simulink model "Xe_Model_Redo_June_26"  (R2018a)
settings: Solver=VariableStepAuto  StartTime=0.0  StopTime=5E5+96*60*60  RelTol=1e-3
values from neighbouring files (symbols this model uses):
  A_pipe = pi*r_pipe^2    (= 0.0126676869774)    [Startup_Script.m]
  alpha_FS = 0.517E-16    (= 5.17e-17)    [Startup_Script.m]
  alpha_G_R1 = 0.334E-17    (= 3.34e-18)    [Startup_Script.m]
  alpha_G_R2 = 0.699E-17    (= 6.99e-18)    [Startup_Script.m]
  alpha_G_R3 = 0.669E-17    (= 6.69e-18)    [Startup_Script.m]
  alpha_G_R4 = 0.791E-18    (= 7.91e-19)    [Startup_Script.m]
  D_g = 2.37E-9    (= 2.37e-09)    [Startup_Script.m]
  epsilon = 0.1    [Startup_Script.m]
  eta_b = 1E-4    (= 0.0001)    [Startup_Script.m]
  eta_fs = 1.2E-4    (= 0.00012)    [Startup_Script.m]
  f_cv = 0.004    [Startup_Script.m]
  FS_Mu_A = 4340    [Startup_Script.m]
  FS_Mu_K = 0.084    [Startup_Script.m]
  FS_Mu_MSRE = 0.007027    [Startup_Script.m]
  FS_rho_A = 3.628    [Startup_Script.m]
  FS_rho_B = 0.00066    [Startup_Script.m]
  FS_rho_MSRE = 2082    [Startup_Script.m]
  gamma_i = 0.0293524    [Startup_Script.m]
  gamma_te = 0.0322482    [Startup_Script.m]
  gamma_xe = 0.00257324    [Startup_Script.m]
  h_fc = 1.6    [Startup_Script.m]
  H_Xe_a = 5.713e-13    [Startup_Script.m]
  H_Xe_b = -7.937e-10    [Startup_Script.m]
  H_Xe_c = 2.809e-07    [Startup_Script.m]
  HX_r_Tube = ((0.5-0.042)/2)*2.54E-2    (= 0.0058166)    [Startup_Script.m]
  HX_XS = HX_N_Tubes*(pi*HX_r_Tube^2)    (= 0.0168999490356)    [Startup_Script.m]
  k_b = 1.3806E-23    (= 1.3806e-23)    [Startup_Script.m]
  lambda_i = 2.9306070546251702E-5    (= 2.93060705463e-05)    [Startup_Script.m]
  lambda_te = 0.036481430555786593    (= 0.0364814305558)    [Startup_Script.m]
  lambda_xe = 2.0924e-05    [Startup_Script.m]
  N_FC_R1 = 12    [Startup_Script.m]
  N_FC_R2 = 940    [Startup_Script.m]
  N_FC_R3 = 108    [Startup_Script.m]
  N_FC_R4 = 78    [Startup_Script.m]
  P_pump = 35420    [Startup_Script.m]
  phi0 = 3.98E+17    (= 3.98e+17)    [Startup_Script.m]
  phi_G_R_1 = mean(interp1(phi_G_R,phi_G_phi, linspace(0,r_g_r1)))    [Startup_Script.m]
  phi_G_R_2 = mean(interp1(phi_G_R,phi_G_phi, linspace(r_g_r1,r_g_r2)))    [Startup_Script.m]
  phi_G_R_3 = mean(interp1(phi_G_R,phi_G_phi, linspace(r_g_r2,r_g_r3)))    [Startup_Script.m]
  phi_G_R_4 = mean(interp1(phi_G_R,phi_G_phi, linspace(r_g_r3,r_g_r4)))    [Startup_Script.m]
  Q_strpr = 0.003155    [Startup_Script.m]
  Q_tot = 0.07571    [Startup_Script.m]
  r_b = 0.000254    [Startup_Script.m]
  r_fc = 0.79e-2    (= 0.0079)    [Startup_Script.m]
  r_pipe = (5E-2*2.54)/2    (= 0.0635)    [Startup_Script.m]
  r_xe = 2.16E-10    (= 2.16e-10)    [Startup_Script.m]
  Re_CA = 25800    [Startup_Script.m]
  Re_LH = 1E4    (= 10000)    [Startup_Script.m]
  Re_UH = 1E4    (= 10000)    [Startup_Script.m]
  sig_a_xe = 1.18E-22    (= 1.18e-22)    [Startup_Script.m]
  Sig_f = 0.15    [Startup_Script.m]
  T_CA_0 = T_INLET    (= 907.594444444)    [Startup_Script.m]
  T_FP_0 = T_OUTLET    (= 935.372222222)    [Startup_Script.m]
  T_FS_R_1_0 = mean(interp1(R_fs_m,T_fs_K, linspace(0,r_g_r1)))    [Startup_Script.m]
  T_FS_R_2_0 = mean(interp1(R_fs_m,T_fs_K, linspace(r_g_r1,r_g_r2)))    [Startup_Script.m]
  T_FS_R_3_0 = mean(interp1(R_fs_m,T_fs_K, linspace(r_g_r2,r_g_r3)))    [Startup_Script.m]
  T_FS_R_4_0 = mean(interp1(R_fs_m,T_fs_K, linspace(r_g_r3,r_g_r4)))    [Startup_Script.m]
  T_G_R_1_0 = mean(interp1(R_gr_m,T_gr_K, linspace(0,r_g_r1)))    [Startup_Script.m]
  T_HX_0 = 0.5*(T_OUTLET + T_INLET)    (= 921.483333333)    [Startup_Script.m]
  T_LH_0 = T_INLET    (= 907.594444444)    [Startup_Script.m]
  T_Mes = 928.15    [Startup_Script.m]
  T_P100_0 = T_OUTLET    (= 935.372222222)    [Startup_Script.m]
  T_P101_0 = T_OUTLET    (= 935.372222222)    [Startup_Script.m]
  T_P102_0 = T_INLET    (= 907.594444444)    [Startup_Script.m]
  T_Salt_0 = 900    [Startup_Script.m]
  T_UH_0 = T_OUTLET    (= 935.372222222)    [Startup_Script.m]
  U_FC_R1 = 0.607    [Startup_Script.m]
  U_FC_R2 = 0.183    [Startup_Script.m]
  U_FC_R3 = 0.454    [Startup_Script.m]
  U_FC_R4 = 0.250    (= 0.25)    [Startup_Script.m]
  V_CA_0 = 9.7*cubed_foot_to_cubed_meter    (= 0.274673445)    [Startup_Script.m]
  V_FP_0 = (0.9+3.2)*cubed_foot_to_cubed_meter    (= 0.116099085)    [Startup_Script.m]
  V_HX_0 = 6.1*cubed_foot_to_cubed_meter    (= 0.172732785)    [Startup_Script.m]
  V_LH_0 = 10.0*cubed_foot_to_cubed_meter    (= 0.2831685)    [Startup_Script.m]
  V_P100_0 = 2.1*cubed_foot_to_cubed_meter    (= 0.059465385)    [Startup_Script.m]
  V_P101_0 = 0.8*cubed_foot_to_cubed_meter    (= 0.02265348)    [Startup_Script.m]
  V_P102_0 = 2.2*cubed_foot_to_cubed_meter    (= 0.06229707)    [Startup_Script.m]
  V_R1_0 = V_Core_FS_0 *N_FC_R1/N_FC_tot    (= 0.00753107712766)    [Startup_Script.m]
  V_R2_0 = V_Core_FS_0 *N_FC_R2/N_FC_tot    (= 0.589934375)    [Startup_Script.m]
  V_R3_0 = V_Core_FS_0 *N_FC_R3/N_FC_tot    (= 0.0677796941489)    [Startup_Script.m]
  V_R4_0 = V_Core_FS_0 *N_FC_R4/N_FC_tot    (= 0.0489520013298)    [Startup_Script.m]
  V_UH_0 = 10.5*cubed_foot_to_cubed_meter    (= 0.297326925)    [Startup_Script.m]
undefined symbols (not defined in the file or in its folder): magnitude, V_CA, V_HX, V_P2, V_P3, V_R1, V_R2, V_R3, V_R4, V_UH
libraries: simulink x4, dspindex x4, dspstat3 x4, SignalEditorBlockLib x2
(part 11 of 11)

== system Xe_Model_Redo_June_26/Bubbles/Bubble Mass Transfer/Bubble Total KMA/KMA_LH/MTC LH/Re_Num  Scaled/Density W Scaling1/Cantor F1 Density1 ==
  note: K -> deg. C
  T_Salt [k] : Inport
  Constant : Constant  Value=FS_rho_A
  Constant1 : Constant  Value=FS_rho_B
  Constant2 : Constant  Value=273.15
  Display : Display
      settings: Format=short_e
  Display1 : Display
  Product : Product
  Sum : Sum  Inputs=|+-
  Sum1 : Sum  Inputs=+-
  "g/cm^3 -> kg/m^3" : Gain  Gain=1000
  rho [kg/m^3] : Outport
  wires:
  Sum/1 -> "g/cm^3 -> kg/m^3"/1
  Product/1 -> Sum/2
  Constant1/1 -> Display/1, Product/1
  "g/cm^3 -> kg/m^3"/1 -> rho [kg/m^3]/1
  Constant/1 -> Display1/1, Sum/1
  T_Salt [k]/1 -> Sum1/1
  Constant2/1 -> Sum1/2
  Sum1/1 -> Product/2

== system Xe_Model_Redo_June_26/Bubbles/Bubble Mass Transfer/Bubble Total KMA/KMA_LH/MTC LH/Re_Num  Scaled/Density W Scaling3/Cantor F1 Density ==
  note: K -> deg. C
  T_Salt [k] : Inport
  Constant : Constant  Value=FS_rho_A
  Constant1 : Constant  Value=FS_rho_B
  Constant2 : Constant  Value=273.15
  Display : Display
      settings: Format=short_e
  Display1 : Display
  Product : Product
  Sum : Sum  Inputs=|+-
  Sum1 : Sum  Inputs=+-
  "g/cm^3 -> kg/m^3" : Gain  Gain=1000
  rho [kg/m^3] : Outport
  wires:
  Sum/1 -> "g/cm^3 -> kg/m^3"/1
  Product/1 -> Sum/2
  Constant1/1 -> Display/1, Product/1
  "g/cm^3 -> kg/m^3"/1 -> rho [kg/m^3]/1
  Constant/1 -> Display1/1, Sum/1
  T_Salt [k]/1 -> Sum1/1
  Constant2/1 -> Sum1/2
  Sum1/1 -> Product/2

== system Xe_Model_Redo_June_26/Bubbles/Bubble Mass Transfer/Bubble Total KMA/KMA_LH/MTC LH/Re_Num  Scaled/Density W Scaling3/Cantor F1 Density1 ==
  note: K -> deg. C
  T_Salt [k] : Inport
  Constant : Constant  Value=FS_rho_A
  Constant1 : Constant  Value=FS_rho_B
  Constant2 : Constant  Value=273.15
  Display : Display
      settings: Format=short_e
  Display1 : Display
  Product : Product
  Sum : Sum  Inputs=|+-
  Sum1 : Sum  Inputs=+-
  "g/cm^3 -> kg/m^3" : Gain  Gain=1000
  rho [kg/m^3] : Outport
  wires:
  Sum/1 -> "g/cm^3 -> kg/m^3"/1
  Product/1 -> Sum/2
  Constant1/1 -> Display/1, Product/1
  "g/cm^3 -> kg/m^3"/1 -> rho [kg/m^3]/1
  Constant/1 -> Display1/1, Sum/1
  T_Salt [k]/1 -> Sum1/1
  Constant2/1 -> Sum1/2
  Sum1/1 -> Product/2

== system Xe_Model_Redo_June_26/Bubbles/Bubble Mass Transfer/Bubble Total KMA/KMA_LH/MTC LH/Re_Num  Scaled/Viscosity W Scaling1/Cantor Viscosity F1 ==
  T_Salt [k] : Inport
  Constant : Constant  Value=FS_Mu_A
  Constant1 : Constant  Value=FS_Mu_K
  Display1 : Display
  Divide : Product  Inputs=*/
  Math Function : Math  SaturateOnIntegerOverflow=on
  Product : Product
  "centipoise -> Pa S" : Gain  Gain=0.001
  Mu [Pa S] : Outport
  wires:
  Constant1/1 -> Product/2
  T_Salt [k]/1 -> Divide/2
  "centipoise -> Pa S"/1 -> Display1/1, Mu [Pa S]/1
  Product/1 -> "centipoise -> Pa S"/1
  Constant/1 -> Divide/1
  Math Function/1 -> Product/1
  Divide/1 -> Math Function/1

== system Xe_Model_Redo_June_26/Bubbles/Bubble Mass Transfer/Bubble Total KMA/KMA_LH/MTC LH/Re_Num  Scaled/Viscosity W Scaling1/Nominal Value for Cantor Viscosity F1 ==
  T_Salt [k] : Inport
  Constant : Constant  Value=FS_Mu_A
  Constant1 : Constant  Value=FS_Mu_K
  Display1 : Display
  Divide : Product  Inputs=*/
  Math Function : Math  SaturateOnIntegerOverflow=on
  Product : Product
  "centipoise -> Pa S" : Gain  Gain=0.001
  Mu [Pa S] : Outport
  wires:
  Constant1/1 -> Product/2
  T_Salt [k]/1 -> Divide/2
  "centipoise -> Pa S"/1 -> Display1/1, Mu [Pa S]/1
  Product/1 -> "centipoise -> Pa S"/1
  Constant/1 -> Divide/1
  Math Function/1 -> Product/1
  Divide/1 -> Math Function/1

== system Xe_Model_Redo_June_26/Bubbles/Bubble Mass Transfer/Bubble Total KMA/KMA_LH/MTC LH/Re_Num  Scaled/Viscosity W Scaling3/Cantor Viscosity F1 ==
  T_Salt [k] : Inport
  Constant : Constant  Value=FS_Mu_A
  Constant1 : Constant  Value=FS_Mu_K
  Display1 : Display
  Divide : Product  Inputs=*/
  Math Function : Math  SaturateOnIntegerOverflow=on
  Product : Product
  "centipoise -> Pa S" : Gain  Gain=0.001
  Mu [Pa S] : Outport
  wires:
  Constant1/1 -> Product/2
  T_Salt [k]/1 -> Divide/2
  "centipoise -> Pa S"/1 -> Display1/1, Mu [Pa S]/1
  Product/1 -> "centipoise -> Pa S"/1
  Constant/1 -> Divide/1
  Math Function/1 -> Product/1
  Divide/1 -> Math Function/1

== system Xe_Model_Redo_June_26/Bubbles/Bubble Mass Transfer/Bubble Total KMA/KMA_LH/MTC LH/Re_Num  Scaled/Viscosity W Scaling3/Nominal Value for Cantor Viscosity F1 ==
  T_Salt [k] : Inport
  Constant : Constant  Value=FS_Mu_A
  Constant1 : Constant  Value=FS_Mu_K
  Display1 : Display
  Divide : Product  Inputs=*/
  Math Function : Math  SaturateOnIntegerOverflow=on
  Product : Product
  "centipoise -> Pa S" : Gain  Gain=0.001
  Mu [Pa S] : Outport
  wires:
  Constant1/1 -> Product/2
  T_Salt [k]/1 -> Divide/2
  "centipoise -> Pa S"/1 -> Display1/1, Mu [Pa S]/1
  Product/1 -> "centipoise -> Pa S"/1
  Constant/1 -> Divide/1
  Math Function/1 -> Product/1
  Divide/1 -> Math Function/1

== system Xe_Model_Redo_June_26/Bubbles/Bubble Mass Transfer/Bubble Total KMA/KMA_UH/MTC UH/Re_Num  Scaled/Density W Scaling1/Cantor F1 Density ==
  note: K -> deg. C
  T_Salt [k] : Inport
  Constant : Constant  Value=FS_rho_A
  Constant1 : Constant  Value=FS_rho_B
  Constant2 : Constant  Value=273.15
  Display : Display
      settings: Format=short_e
  Display1 : Display
  Product : Product
  Sum : Sum  Inputs=|+-
  Sum1 : Sum  Inputs=+-
  "g/cm^3 -> kg/m^3" : Gain  Gain=1000
  rho [kg/m^3] : Outport
  wires:
  Sum/1 -> "g/cm^3 -> kg/m^3"/1
  Product/1 -> Sum/2
  Constant1/1 -> Display/1, Product/1
  "g/cm^3 -> kg/m^3"/1 -> rho [kg/m^3]/1
  Constant/1 -> Display1/1, Sum/1
  T_Salt [k]/1 -> Sum1/1
  Constant2/1 -> Sum1/2
  Sum1/1 -> Product/2

== system Xe_Model_Redo_June_26/Bubbles/Bubble Mass Transfer/Bubble Total KMA/KMA_UH/MTC UH/Re_Num  Scaled/Density W Scaling1/Cantor F1 Density1 ==
  note: K -> deg. C
  T_Salt [k] : Inport
  Constant : Constant  Value=FS_rho_A
  Constant1 : Constant  Value=FS_rho_B
  Constant2 : Constant  Value=273.15
  Display : Display
      settings: Format=short_e
  Display1 : Display
  Product : Product
  Sum : Sum  Inputs=|+-
  Sum1 : Sum  Inputs=+-
  "g/cm^3 -> kg/m^3" : Gain  Gain=1000
  rho [kg/m^3] : Outport
  wires:
  Sum/1 -> "g/cm^3 -> kg/m^3"/1
  Product/1 -> Sum/2
  Constant1/1 -> Display/1, Product/1
  "g/cm^3 -> kg/m^3"/1 -> rho [kg/m^3]/1
  Constant/1 -> Display1/1, Sum/1
  T_Salt [k]/1 -> Sum1/1
  Constant2/1 -> Sum1/2
  Sum1/1 -> Product/2

== system Xe_Model_Redo_June_26/Bubbles/Bubble Mass Transfer/Bubble Total KMA/KMA_UH/MTC UH/Re_Num  Scaled/Density W Scaling3/Cantor F1 Density ==
  note: K -> deg. C
  T_Salt [k] : Inport
  Constant : Constant  Value=FS_rho_A
  Constant1 : Constant  Value=FS_rho_B
  Constant2 : Constant  Value=273.15
  Display : Display
      settings: Format=short_e
  Display1 : Display
  Product : Product
  Sum : Sum  Inputs=|+-
  Sum1 : Sum  Inputs=+-
  "g/cm^3 -> kg/m^3" : Gain  Gain=1000
  rho [kg/m^3] : Outport
  wires:
  Sum/1 -> "g/cm^3 -> kg/m^3"/1
  Product/1 -> Sum/2
  Constant1/1 -> Display/1, Product/1
  "g/cm^3 -> kg/m^3"/1 -> rho [kg/m^3]/1
  Constant/1 -> Display1/1, Sum/1
  T_Salt [k]/1 -> Sum1/1
  Constant2/1 -> Sum1/2
  Sum1/1 -> Product/2

== system Xe_Model_Redo_June_26/Bubbles/Bubble Mass Transfer/Bubble Total KMA/KMA_UH/MTC UH/Re_Num  Scaled/Density W Scaling3/Cantor F1 Density1 ==
  note: K -> deg. C
  T_Salt [k] : Inport
  Constant : Constant  Value=FS_rho_A
  Constant1 : Constant  Value=FS_rho_B
  Constant2 : Constant  Value=273.15
  Display : Display
      settings: Format=short_e
  Display1 : Display
  Product : Product
  Sum : Sum  Inputs=|+-
  Sum1 : Sum  Inputs=+-
  "g/cm^3 -> kg/m^3" : Gain  Gain=1000
  rho [kg/m^3] : Outport
  wires:
  Sum/1 -> "g/cm^3 -> kg/m^3"/1
  Product/1 -> Sum/2
  Constant1/1 -> Display/1, Product/1
  "g/cm^3 -> kg/m^3"/1 -> rho [kg/m^3]/1
  Constant/1 -> Display1/1, Sum/1
  T_Salt [k]/1 -> Sum1/1
  Constant2/1 -> Sum1/2
  Sum1/1 -> Product/2

== system Xe_Model_Redo_June_26/Bubbles/Bubble Mass Transfer/Bubble Total KMA/KMA_UH/MTC UH/Re_Num  Scaled/Viscosity W Scaling1/Cantor Viscosity F1 ==
  T_Salt [k] : Inport
  Constant : Constant  Value=FS_Mu_A
  Constant1 : Constant  Value=FS_Mu_K
  Display1 : Display
  Divide : Product  Inputs=*/
  Math Function : Math  SaturateOnIntegerOverflow=on
  Product : Product
  "centipoise -> Pa S" : Gain  Gain=0.001
  Mu [Pa S] : Outport
  wires:
  Constant1/1 -> Product/2
  T_Salt [k]/1 -> Divide/2
  "centipoise -> Pa S"/1 -> Display1/1, Mu [Pa S]/1
  Product/1 -> "centipoise -> Pa S"/1
  Constant/1 -> Divide/1
  Math Function/1 -> Product/1
  Divide/1 -> Math Function/1

== system Xe_Model_Redo_June_26/Bubbles/Bubble Mass Transfer/Bubble Total KMA/KMA_UH/MTC UH/Re_Num  Scaled/Viscosity W Scaling1/Nominal Value for Cantor Viscosity F1 ==
  T_Salt [k] : Inport
  Constant : Constant  Value=FS_Mu_A
  Constant1 : Constant  Value=FS_Mu_K
  Display1 : Display
  Divide : Product  Inputs=*/
  Math Function : Math  SaturateOnIntegerOverflow=on
  Product : Product
  "centipoise -> Pa S" : Gain  Gain=0.001
  Mu [Pa S] : Outport
  wires:
  Constant1/1 -> Product/2
  T_Salt [k]/1 -> Divide/2
  "centipoise -> Pa S"/1 -> Display1/1, Mu [Pa S]/1
  Product/1 -> "centipoise -> Pa S"/1
  Constant/1 -> Divide/1
  Math Function/1 -> Product/1
  Divide/1 -> Math Function/1

== system Xe_Model_Redo_June_26/Bubbles/Bubble Mass Transfer/Bubble Total KMA/KMA_UH/MTC UH/Re_Num  Scaled/Viscosity W Scaling3/Cantor Viscosity F1 ==
  T_Salt [k] : Inport
  Constant : Constant  Value=FS_Mu_A
  Constant1 : Constant  Value=FS_Mu_K
  Display1 : Display
  Divide : Product  Inputs=*/
  Math Function : Math  SaturateOnIntegerOverflow=on
  Product : Product
  "centipoise -> Pa S" : Gain  Gain=0.001
  Mu [Pa S] : Outport
  wires:
  Constant1/1 -> Product/2
  T_Salt [k]/1 -> Divide/2
  "centipoise -> Pa S"/1 -> Display1/1, Mu [Pa S]/1
  Product/1 -> "centipoise -> Pa S"/1
  Constant/1 -> Divide/1
  Math Function/1 -> Product/1
  Divide/1 -> Math Function/1

== system Xe_Model_Redo_June_26/Bubbles/Bubble Mass Transfer/Bubble Total KMA/KMA_UH/MTC UH/Re_Num  Scaled/Viscosity W Scaling3/Nominal Value for Cantor Viscosity F1 ==
  T_Salt [k] : Inport
  Constant : Constant  Value=FS_Mu_A
  Constant1 : Constant  Value=FS_Mu_K
  Display1 : Display
  Divide : Product  Inputs=*/
  Math Function : Math  SaturateOnIntegerOverflow=on
  Product : Product
  "centipoise -> Pa S" : Gain  Gain=0.001
  Mu [Pa S] : Outport
  wires:
  Constant1/1 -> Product/2
  T_Salt [k]/1 -> Divide/2
  "centipoise -> Pa S"/1 -> Display1/1, Mu [Pa S]/1
  Product/1 -> "centipoise -> Pa S"/1
  Constant/1 -> Divide/1
  Math Function/1 -> Product/1
  Divide/1 -> Math Function/1

== system Xe_Model_Redo_June_26/Bubbles/Bubble Mass Transfer/CA/KMA_CA/CA  MTC/Re_Num  Scaled/Density W Scaling1/Cantor F1 Density ==
  note: K -> deg. C
  T_Salt [k] : Inport
  Constant : Constant  Value=FS_rho_A
  Constant1 : Constant  Value=FS_rho_B
  Constant2 : Constant  Value=273.15
  Display : Display
      settings: Format=short_e
  Display1 : Display
  Product : Product
  Sum : Sum  Inputs=|+-
  Sum1 : Sum  Inputs=+-
  "g/cm^3 -> kg/m^3" : Gain  Gain=1000
  rho [kg/m^3] : Outport
  wires:
  Sum/1 -> "g/cm^3 -> kg/m^3"/1
  Product/1 -> Sum/2
  Constant1/1 -> Display/1, Product/1
  "g/cm^3 -> kg/m^3"/1 -> rho [kg/m^3]/1
  Constant/1 -> Display1/1, Sum/1
  T_Salt [k]/1 -> Sum1/1
  Constant2/1 -> Sum1/2
  Sum1/1 -> Product/2

== system Xe_Model_Redo_June_26/Bubbles/Bubble Mass Transfer/CA/KMA_CA/CA  MTC/Re_Num  Scaled/Density W Scaling1/Cantor F1 Density1 ==
  note: K -> deg. C
  T_Salt [k] : Inport
  Constant : Constant  Value=FS_rho_A
  Constant1 : Constant  Value=FS_rho_B
  Constant2 : Constant  Value=273.15
  Display : Display
      settings: Format=short_e
  Display1 : Display
  Product : Product
  Sum : Sum  Inputs=|+-
  Sum1 : Sum  Inputs=+-
  "g/cm^3 -> kg/m^3" : Gain  Gain=1000
  rho [kg/m^3] : Outport
  wires:
  Sum/1 -> "g/cm^3 -> kg/m^3"/1
  Product/1 -> Sum/2
  Constant1/1 -> Display/1, Product/1
  "g/cm^3 -> kg/m^3"/1 -> rho [kg/m^3]/1
  Constant/1 -> Display1/1, Sum/1
  T_Salt [k]/1 -> Sum1/1
  Constant2/1 -> Sum1/2
  Sum1/1 -> Product/2

== system Xe_Model_Redo_June_26/Bubbles/Bubble Mass Transfer/CA/KMA_CA/CA  MTC/Re_Num  Scaled/Density W Scaling3/Cantor F1 Density ==
  note: K -> deg. C
  T_Salt [k] : Inport
  Constant : Constant  Value=FS_rho_A
  Constant1 : Constant  Value=FS_rho_B
  Constant2 : Constant  Value=273.15
  Display : Display
      settings: Format=short_e
  Display1 : Display
  Product : Product
  Sum : Sum  Inputs=|+-
  Sum1 : Sum  Inputs=+-
  "g/cm^3 -> kg/m^3" : Gain  Gain=1000
  rho [kg/m^3] : Outport
  wires:
  Sum/1 -> "g/cm^3 -> kg/m^3"/1
  Product/1 -> Sum/2
  Constant1/1 -> Display/1, Product/1
  "g/cm^3 -> kg/m^3"/1 -> rho [kg/m^3]/1
  Constant/1 -> Display1/1, Sum/1
  T_Salt [k]/1 -> Sum1/1
  Constant2/1 -> Sum1/2
  Sum1/1 -> Product/2

== system Xe_Model_Redo_June_26/Bubbles/Bubble Mass Transfer/CA/KMA_CA/CA  MTC/Re_Num  Scaled/Density W Scaling3/Cantor F1 Density1 ==
  note: K -> deg. C
  T_Salt [k] : Inport
  Constant : Constant  Value=FS_rho_A
  Constant1 : Constant  Value=FS_rho_B
  Constant2 : Constant  Value=273.15
  Display : Display
      settings: Format=short_e
  Display1 : Display
  Product : Product
  Sum : Sum  Inputs=|+-
  Sum1 : Sum  Inputs=+-
  "g/cm^3 -> kg/m^3" : Gain  Gain=1000
  rho [kg/m^3] : Outport
  wires:
  Sum/1 -> "g/cm^3 -> kg/m^3"/1
  Product/1 -> Sum/2
  Constant1/1 -> Display/1, Product/1
  "g/cm^3 -> kg/m^3"/1 -> rho [kg/m^3]/1
  Constant/1 -> Display1/1, Sum/1
  T_Salt [k]/1 -> Sum1/1
  Constant2/1 -> Sum1/2
  Sum1/1 -> Product/2

== system Xe_Model_Redo_June_26/Bubbles/Bubble Mass Transfer/CA/KMA_CA/CA  MTC/Re_Num  Scaled/Viscosity W Scaling1/Cantor Viscosity F1 ==
  T_Salt [k] : Inport
  Constant : Constant  Value=FS_Mu_A
  Constant1 : Constant  Value=FS_Mu_K
  Display1 : Display
  Divide : Product  Inputs=*/
  Math Function : Math  SaturateOnIntegerOverflow=on
  Product : Product
  "centipoise -> Pa S" : Gain  Gain=0.001
  Mu [Pa S] : Outport
  wires:
  Constant1/1 -> Product/2
  T_Salt [k]/1 -> Divide/2
  "centipoise -> Pa S"/1 -> Display1/1, Mu [Pa S]/1
  Product/1 -> "centipoise -> Pa S"/1
  Constant/1 -> Divide/1
  Math Function/1 -> Product/1
  Divide/1 -> Math Function/1

== system Xe_Model_Redo_June_26/Bubbles/Bubble Mass Transfer/CA/KMA_CA/CA  MTC/Re_Num  Scaled/Viscosity W Scaling1/Nominal Value for Cantor Viscosity F1 ==
  T_Salt [k] : Inport
  Constant : Constant  Value=FS_Mu_A
  Constant1 : Constant  Value=FS_Mu_K
  Display1 : Display
  Divide : Product  Inputs=*/
  Math Function : Math  SaturateOnIntegerOverflow=on
  Product : Product
  "centipoise -> Pa S" : Gain  Gain=0.001
  Mu [Pa S] : Outport
  wires:
  Constant1/1 -> Product/2
  T_Salt [k]/1 -> Divide/2
  "centipoise -> Pa S"/1 -> Display1/1, Mu [Pa S]/1
  Product/1 -> "centipoise -> Pa S"/1
  Constant/1 -> Divide/1
  Math Function/1 -> Product/1
  Divide/1 -> Math Function/1

== system Xe_Model_Redo_June_26/Bubbles/Bubble Mass Transfer/CA/KMA_CA/CA  MTC/Re_Num  Scaled/Viscosity W Scaling3/Cantor Viscosity F1 ==
  T_Salt [k] : Inport
  Constant : Constant  Value=FS_Mu_A
  Constant1 : Constant  Value=FS_Mu_K
  Display1 : Display
  Divide : Product  Inputs=*/
  Math Function : Math  SaturateOnIntegerOverflow=on
  Product : Product
  "centipoise -> Pa S" : Gain  Gain=0.001
  Mu [Pa S] : Outport
  wires:
  Constant1/1 -> Product/2
  T_Salt [k]/1 -> Divide/2
  "centipoise -> Pa S"/1 -> Display1/1, Mu [Pa S]/1
  Product/1 -> "centipoise -> Pa S"/1
  Constant/1 -> Divide/1
  Math Function/1 -> Product/1
  Divide/1 -> Math Function/1

== system Xe_Model_Redo_June_26/Bubbles/Bubble Mass Transfer/CA/KMA_CA/CA  MTC/Re_Num  Scaled/Viscosity W Scaling3/Nominal Value for Cantor Viscosity F1 ==
  T_Salt [k] : Inport
  Constant : Constant  Value=FS_Mu_A
  Constant1 : Constant  Value=FS_Mu_K
  Display1 : Display
  Divide : Product  Inputs=*/
  Math Function : Math  SaturateOnIntegerOverflow=on
  Product : Product
  "centipoise -> Pa S" : Gain  Gain=0.001
  Mu [Pa S] : Outport
  wires:
  Constant1/1 -> Product/2
  T_Salt [k]/1 -> Divide/2
  "centipoise -> Pa S"/1 -> Display1/1, Mu [Pa S]/1
  Product/1 -> "centipoise -> Pa S"/1
  Constant/1 -> Divide/1
  Math Function/1 -> Product/1
  Divide/1 -> Math Function/1

== system Xe_Model_Redo_June_26/Bubbles/Bubble Mass Transfer/LH/KMA_LH/MTC LH/Re_Num  Scaled/Density W Scaling1/Cantor F1 Density ==
  note: K -> deg. C
  T_Salt [k] : Inport
  Constant : Constant  Value=FS_rho_A
  Constant1 : Constant  Value=FS_rho_B
  Constant2 : Constant  Value=273.15
  Display : Display
      settings: Format=short_e
  Display1 : Display
  Product : Product
  Sum : Sum  Inputs=|+-
  Sum1 : Sum  Inputs=+-
  "g/cm^3 -> kg/m^3" : Gain  Gain=1000
  rho [kg/m^3] : Outport
  wires:
  Sum/1 -> "g/cm^3 -> kg/m^3"/1
  Product/1 -> Sum/2
  Constant1/1 -> Display/1, Product/1
  "g/cm^3 -> kg/m^3"/1 -> rho [kg/m^3]/1
  Constant/1 -> Display1/1, Sum/1
  T_Salt [k]/1 -> Sum1/1
  Constant2/1 -> Sum1/2
  Sum1/1 -> Product/2

== system Xe_Model_Redo_June_26/Bubbles/Bubble Mass Transfer/LH/KMA_LH/MTC LH/Re_Num  Scaled/Density W Scaling1/Cantor F1 Density1 ==
  note: K -> deg. C
  T_Salt [k] : Inport
  Constant : Constant  Value=FS_rho_A
  Constant1 : Constant  Value=FS_rho_B
  Constant2 : Constant  Value=273.15
  Display : Display
      settings: Format=short_e
  Display1 : Display
  Product : Product
  Sum : Sum  Inputs=|+-
  Sum1 : Sum  Inputs=+-
  "g/cm^3 -> kg/m^3" : Gain  Gain=1000
  rho [kg/m^3] : Outport
  wires:
  Sum/1 -> "g/cm^3 -> kg/m^3"/1
  Product/1 -> Sum/2
  Constant1/1 -> Display/1, Product/1
  "g/cm^3 -> kg/m^3"/1 -> rho [kg/m^3]/1
  Constant/1 -> Display1/1, Sum/1
  T_Salt [k]/1 -> Sum1/1
  Constant2/1 -> Sum1/2
  Sum1/1 -> Product/2

== system Xe_Model_Redo_June_26/Bubbles/Bubble Mass Transfer/LH/KMA_LH/MTC LH/Re_Num  Scaled/Density W Scaling3/Cantor F1 Density ==
  note: K -> deg. C
  T_Salt [k] : Inport
  Constant : Constant  Value=FS_rho_A
  Constant1 : Constant  Value=FS_rho_B
  Constant2 : Constant  Value=273.15
  Display : Display
      settings: Format=short_e
  Display1 : Display
  Product : Product
  Sum : Sum  Inputs=|+-
  Sum1 : Sum  Inputs=+-
  "g/cm^3 -> kg/m^3" : Gain  Gain=1000
  rho [kg/m^3] : Outport
  wires:
  Sum/1 -> "g/cm^3 -> kg/m^3"/1
  Product/1 -> Sum/2
  Constant1/1 -> Display/1, Product/1
  "g/cm^3 -> kg/m^3"/1 -> rho [kg/m^3]/1
  Constant/1 -> Display1/1, Sum/1
  T_Salt [k]/1 -> Sum1/1
  Constant2/1 -> Sum1/2
  Sum1/1 -> Product/2

== system Xe_Model_Redo_June_26/Bubbles/Bubble Mass Transfer/LH/KMA_LH/MTC LH/Re_Num  Scaled/Density W Scaling3/Cantor F1 Density1 ==
  note: K -> deg. C
  T_Salt [k] : Inport
  Constant : Constant  Value=FS_rho_A
  Constant1 : Constant  Value=FS_rho_B
  Constant2 : Constant  Value=273.15
  Display : Display
      settings: Format=short_e
  Display1 : Display
  Product : Product
  Sum : Sum  Inputs=|+-
  Sum1 : Sum  Inputs=+-
  "g/cm^3 -> kg/m^3" : Gain  Gain=1000
  rho [kg/m^3] : Outport
  wires:
  Sum/1 -> "g/cm^3 -> kg/m^3"/1
  Product/1 -> Sum/2
  Constant1/1 -> Display/1, Product/1
  "g/cm^3 -> kg/m^3"/1 -> rho [kg/m^3]/1
  Constant/1 -> Display1/1, Sum/1
  T_Salt [k]/1 -> Sum1/1
  Constant2/1 -> Sum1/2
  Sum1/1 -> Product/2

== system Xe_Model_Redo_June_26/Bubbles/Bubble Mass Transfer/LH/KMA_LH/MTC LH/Re_Num  Scaled/Viscosity W Scaling1/Cantor Viscosity F1 ==
  T_Salt [k] : Inport
  Constant : Constant  Value=FS_Mu_A
  Constant1 : Constant  Value=FS_Mu_K
  Display1 : Display
  Divide : Product  Inputs=*/
  Math Function : Math  SaturateOnIntegerOverflow=on
  Product : Product
  "centipoise -> Pa S" : Gain  Gain=0.001
  Mu [Pa S] : Outport
  wires:
  Constant1/1 -> Product/2
  T_Salt [k]/1 -> Divide/2
  "centipoise -> Pa S"/1 -> Display1/1, Mu [Pa S]/1
  Product/1 -> "centipoise -> Pa S"/1
  Constant/1 -> Divide/1
  Math Function/1 -> Product/1
  Divide/1 -> Math Function/1

== system Xe_Model_Redo_June_26/Bubbles/Bubble Mass Transfer/LH/KMA_LH/MTC LH/Re_Num  Scaled/Viscosity W Scaling1/Nominal Value for Cantor Viscosity F1 ==
  T_Salt [k] : Inport
  Constant : Constant  Value=FS_Mu_A
  Constant1 : Constant  Value=FS_Mu_K
  Display1 : Display
  Divide : Product  Inputs=*/
  Math Function : Math  SaturateOnIntegerOverflow=on
  Product : Product
  "centipoise -> Pa S" : Gain  Gain=0.001
  Mu [Pa S] : Outport
  wires:
  Constant1/1 -> Product/2
  T_Salt [k]/1 -> Divide/2
  "centipoise -> Pa S"/1 -> Display1/1, Mu [Pa S]/1
  Product/1 -> "centipoise -> Pa S"/1
  Constant/1 -> Divide/1
  Math Function/1 -> Product/1
  Divide/1 -> Math Function/1

== system Xe_Model_Redo_June_26/Bubbles/Bubble Mass Transfer/LH/KMA_LH/MTC LH/Re_Num  Scaled/Viscosity W Scaling3/Cantor Viscosity F1 ==
  T_Salt [k] : Inport
  Constant : Constant  Value=FS_Mu_A
  Constant1 : Constant  Value=FS_Mu_K
  Display1 : Display
  Divide : Product  Inputs=*/
  Math Function : Math  SaturateOnIntegerOverflow=on
  Product : Product
  "centipoise -> Pa S" : Gain  Gain=0.001
  Mu [Pa S] : Outport
  wires:
  Constant1/1 -> Product/2
  T_Salt [k]/1 -> Divide/2
  "centipoise -> Pa S"/1 -> Display1/1, Mu [Pa S]/1
  Product/1 -> "centipoise -> Pa S"/1
  Constant/1 -> Divide/1
  Math Function/1 -> Product/1
  Divide/1 -> Math Function/1

== system Xe_Model_Redo_June_26/Bubbles/Bubble Mass Transfer/LH/KMA_LH/MTC LH/Re_Num  Scaled/Viscosity W Scaling3/Nominal Value for Cantor Viscosity F1 ==
  T_Salt [k] : Inport
  Constant : Constant  Value=FS_Mu_A
  Constant1 : Constant  Value=FS_Mu_K
  Display1 : Display
  Divide : Product  Inputs=*/
  Math Function : Math  SaturateOnIntegerOverflow=on
  Product : Product
  "centipoise -> Pa S" : Gain  Gain=0.001
  Mu [Pa S] : Outport
  wires:
  Constant1/1 -> Product/2
  T_Salt [k]/1 -> Divide/2
  "centipoise -> Pa S"/1 -> Display1/1, Mu [Pa S]/1
  Product/1 -> "centipoise -> Pa S"/1
  Constant/1 -> Divide/1
  Math Function/1 -> Product/1
  Divide/1 -> Math Function/1

== system Xe_Model_Redo_June_26/Bubbles/Bubble Mass Transfer/UH/KMA_UH/MTC UH/Re_Num  Scaled/Density W Scaling1/Cantor F1 Density ==
  note: K -> deg. C
  T_Salt [k] : Inport
  Constant : Constant  Value=FS_rho_A
  Constant1 : Constant  Value=FS_rho_B
  Constant2 : Constant  Value=273.15
  Display : Display
      settings: Format=short_e
  Display1 : Display
  Product : Product
  Sum : Sum  Inputs=|+-
  Sum1 : Sum  Inputs=+-
  "g/cm^3 -> kg/m^3" : Gain  Gain=1000
  rho [kg/m^3] : Outport
  wires:
  Sum/1 -> "g/cm^3 -> kg/m^3"/1
  Product/1 -> Sum/2
  Constant1/1 -> Display/1, Product/1
  "g/cm^3 -> kg/m^3"/1 -> rho [kg/m^3]/1
  Constant/1 -> Display1/1, Sum/1
  T_Salt [k]/1 -> Sum1/1
  Constant2/1 -> Sum1/2
  Sum1/1 -> Product/2

== system Xe_Model_Redo_June_26/Bubbles/Bubble Mass Transfer/UH/KMA_UH/MTC UH/Re_Num  Scaled/Density W Scaling1/Cantor F1 Density1 ==
  note: K -> deg. C
  T_Salt [k] : Inport
  Constant : Constant  Value=FS_rho_A
  Constant1 : Constant  Value=FS_rho_B
  Constant2 : Constant  Value=273.15
  Display : Display
      settings: Format=short_e
  Display1 : Display
  Product : Product
  Sum : Sum  Inputs=|+-
  Sum1 : Sum  Inputs=+-
  "g/cm^3 -> kg/m^3" : Gain  Gain=1000
  rho [kg/m^3] : Outport
  wires:
  Sum/1 -> "g/cm^3 -> kg/m^3"/1
  Product/1 -> Sum/2
  Constant1/1 -> Display/1, Product/1
  "g/cm^3 -> kg/m^3"/1 -> rho [kg/m^3]/1
  Constant/1 -> Display1/1, Sum/1
  T_Salt [k]/1 -> Sum1/1
  Constant2/1 -> Sum1/2
  Sum1/1 -> Product/2

== system Xe_Model_Redo_June_26/Bubbles/Bubble Mass Transfer/UH/KMA_UH/MTC UH/Re_Num  Scaled/Density W Scaling3/Cantor F1 Density ==
  note: K -> deg. C
  T_Salt [k] : Inport
  Constant : Constant  Value=FS_rho_A
  Constant1 : Constant  Value=FS_rho_B
  Constant2 : Constant  Value=273.15
  Display : Display
      settings: Format=short_e
  Display1 : Display
  Product : Product
  Sum : Sum  Inputs=|+-
  Sum1 : Sum  Inputs=+-
  "g/cm^3 -> kg/m^3" : Gain  Gain=1000
  rho [kg/m^3] : Outport
  wires:
  Sum/1 -> "g/cm^3 -> kg/m^3"/1
  Product/1 -> Sum/2
  Constant1/1 -> Display/1, Product/1
  "g/cm^3 -> kg/m^3"/1 -> rho [kg/m^3]/1
  Constant/1 -> Display1/1, Sum/1
  T_Salt [k]/1 -> Sum1/1
  Constant2/1 -> Sum1/2
  Sum1/1 -> Product/2

== system Xe_Model_Redo_June_26/Bubbles/Bubble Mass Transfer/UH/KMA_UH/MTC UH/Re_Num  Scaled/Density W Scaling3/Cantor F1 Density1 ==
  note: K -> deg. C
  T_Salt [k] : Inport
  Constant : Constant  Value=FS_rho_A
  Constant1 : Constant  Value=FS_rho_B
  Constant2 : Constant  Value=273.15
  Display : Display
      settings: Format=short_e
  Display1 : Display
  Product : Product
  Sum : Sum  Inputs=|+-
  Sum1 : Sum  Inputs=+-
  "g/cm^3 -> kg/m^3" : Gain  Gain=1000
  rho [kg/m^3] : Outport
  wires:
  Sum/1 -> "g/cm^3 -> kg/m^3"/1
  Product/1 -> Sum/2
  Constant1/1 -> Display/1, Product/1
  "g/cm^3 -> kg/m^3"/1 -> rho [kg/m^3]/1
  Constant/1 -> Display1/1, Sum/1
  T_Salt [k]/1 -> Sum1/1
  Constant2/1 -> Sum1/2
  Sum1/1 -> Product/2

== system Xe_Model_Redo_June_26/Bubbles/Bubble Mass Transfer/UH/KMA_UH/MTC UH/Re_Num  Scaled/Viscosity W Scaling1/Cantor Viscosity F1 ==
  T_Salt [k] : Inport
  Constant : Constant  Value=FS_Mu_A
  Constant1 : Constant  Value=FS_Mu_K
  Display1 : Display
  Divide : Product  Inputs=*/
  Math Function : Math  SaturateOnIntegerOverflow=on
  Product : Product
  "centipoise -> Pa S" : Gain  Gain=0.001
  Mu [Pa S] : Outport
  wires:
  Constant1/1 -> Product/2
  T_Salt [k]/1 -> Divide/2
  "centipoise -> Pa S"/1 -> Display1/1, Mu [Pa S]/1
  Product/1 -> "centipoise -> Pa S"/1
  Constant/1 -> Divide/1
  Math Function/1 -> Product/1
  Divide/1 -> Math Function/1

== system Xe_Model_Redo_June_26/Bubbles/Bubble Mass Transfer/UH/KMA_UH/MTC UH/Re_Num  Scaled/Viscosity W Scaling1/Nominal Value for Cantor Viscosity F1 ==
  T_Salt [k] : Inport
  Constant : Constant  Value=FS_Mu_A
  Constant1 : Constant  Value=FS_Mu_K
  Display1 : Display
  Divide : Product  Inputs=*/
  Math Function : Math  SaturateOnIntegerOverflow=on
  Product : Product
  "centipoise -> Pa S" : Gain  Gain=0.001
  Mu [Pa S] : Outport
  wires:
  Constant1/1 -> Product/2
  T_Salt [k]/1 -> Divide/2
  "centipoise -> Pa S"/1 -> Display1/1, Mu [Pa S]/1
  Product/1 -> "centipoise -> Pa S"/1
  Constant/1 -> Divide/1
  Math Function/1 -> Product/1
  Divide/1 -> Math Function/1

== system Xe_Model_Redo_June_26/Bubbles/Bubble Mass Transfer/UH/KMA_UH/MTC UH/Re_Num  Scaled/Viscosity W Scaling3/Cantor Viscosity F1 ==
  T_Salt [k] : Inport
  Constant : Constant  Value=FS_Mu_A
  Constant1 : Constant  Value=FS_Mu_K
  Display1 : Display
  Divide : Product  Inputs=*/
  Math Function : Math  SaturateOnIntegerOverflow=on
  Product : Product
  "centipoise -> Pa S" : Gain  Gain=0.001
  Mu [Pa S] : Outport
  wires:
  Constant1/1 -> Product/2
  T_Salt [k]/1 -> Divide/2
  "centipoise -> Pa S"/1 -> Display1/1, Mu [Pa S]/1
  Product/1 -> "centipoise -> Pa S"/1
  Constant/1 -> Divide/1
  Math Function/1 -> Product/1
  Divide/1 -> Math Function/1

== system Xe_Model_Redo_June_26/Bubbles/Bubble Mass Transfer/UH/KMA_UH/MTC UH/Re_Num  Scaled/Viscosity W Scaling3/Nominal Value for Cantor Viscosity F1 ==
  T_Salt [k] : Inport
  Constant : Constant  Value=FS_Mu_A
  Constant1 : Constant  Value=FS_Mu_K
  Display1 : Display
  Divide : Product  Inputs=*/
  Math Function : Math  SaturateOnIntegerOverflow=on
  Product : Product
  "centipoise -> Pa S" : Gain  Gain=0.001
  Mu [Pa S] : Outport
  wires:
  Constant1/1 -> Product/2
  T_Salt [k]/1 -> Divide/2
  "centipoise -> Pa S"/1 -> Display1/1, Mu [Pa S]/1
  Product/1 -> "centipoise -> Pa S"/1
  Constant/1 -> Divide/1
  Math Function/1 -> Product/1
  Divide/1 -> Math Function/1

== matlab function Xe_Model_Redo_June_26/Graphite /Graphite Region 3/Graphite Stringer/Generate FDM Matrix  ==
  data: FDM output; HMat output; BMat output; r0 input; D_g input; epsilon input; rGhost output
function [FDM,HMat,BMat,rGhost]= genMat(r0,D_g,epsilon)

%SETTINGS
%Don't forget to change the value in the blocks:
%%INJECTION VECTOR
%%RHS IDX
nNode = 20;
%%%%%%

%#codegen

%r0 = 0.01454; %graphite stringer radius
dr = r0/(nNode-1); %we have nNode-1 internal 'posts'
rVec = horzcat(linspace(0,r0 ,nNode),r0+dr); %positions of each node, include ghost node
FDM = zeros(nNode+1);

%D_g = 2.37E-9;
%epsilon = 0.1;

A= D_g/epsilon;
 

topRow = zeros(1,nNode+1);
topRow(1) = - (5*A) / (4*dr^2);
topRow(2) = A / dr^2;
topRow(3) = A / (4*dr^2);

FDM(1,:) = topRow; %From Prior Code`

%Second Row
secondRow = zeros(1,nNode+1);

secondRow(1) = A/dr^2 - A/3/dr/rVec(2);
secondRow(2) = - 2*A/dr^2 - A/2/dr/rVec(2);
secondRow(3) = -A/dr^2 + A/dr/rVec(2);
secondRow(4) = -A /dr^2 + A/dr/rVec(2);
secondRow(5) = A/6/dr/rVec(2);

FDM(2,:) = secondRow; %Checked

for idx = 3: (nNode+1)-2
   FDM(idx,idx-2:idx+2) = genRow(idx,A,rVec,dr);
end


%Second Last Row //this is the neumann condition
SLRow = zeros(1,5);
SLRow(1) = -A/12/dr^2 - A/12/dr/rVec(end-1); %need to subtract 2 to account
SLRow(2) = A/3/dr^2 + A/2/dr/rVec(end-1);
SLRow(3) = A/2/dr^2 - 3*A/2/dr/rVec(end-1);
SLRow(4) = - 5*A/3/dr^2 + 5*A/6/dr/rVec(end-1);
SLRow(5) = 11*A/12/dr^2 + A/4/dr/rVec(end-1); %chedcked, sums to zero; checked against mathematica
FDM(end-1,end-4:end) = SLRow;

%Last Row
lastRow = zeros(1,5);
lastRow(1) = -A/12/dr^2;
lastRow(2) = A/3/dr^2;
lastRow(3) = A/2/dr^2;
lastRow(4) = - 5*A/3/dr^2;% - H*R*T*km/epsilon/rVec(end);
lastRow(5) = 11*A/12/dr^2;
FDM(end,end-4:end) = lastRow;

BMat = zeros(nNode+1);
BMat(1:nNode,1:nNode) = eye(nNode);
BMat(end,end-1) = 1;


HMat = zeros(nNode+1);
HMat(end,end-1) = 1;
rGhost = rVec(end);

== matlab function Xe_Model_Redo_June_26/Graphite /Graphite Region 4/Graphite Stringer/Generate FDM Matrix  ==
  data: FDM output; HMat output; BMat output; r0 input; D_g input; epsilon input; rGhost output
function [FDM,HMat,BMat,rGhost]= genMat(r0,D_g,epsilon)

%SETTINGS
%Don't forget to change the value in the blocks:
%%INJECTION VECTOR
%%RHS IDX
nNode = 20;
%%%%%%

%#codegen

%r0 = 0.01454; %graphite stringer radius
dr = r0/(nNode-1); %we have nNode-1 internal 'posts'
rVec = horzcat(linspace(0,r0 ,nNode),r0+dr); %positions of each node, include ghost node
FDM = zeros(nNode+1);

%D_g = 2.37E-9;
%epsilon = 0.1;

A= D_g/epsilon;
 

topRow = zeros(1,nNode+1);
topRow(1) = - (5*A) / (4*dr^2);
topRow(2) = A / dr^2;
topRow(3) = A / (4*dr^2);

FDM(1,:) = topRow; %From Prior Code`

%Second Row
secondRow = zeros(1,nNode+1);

secondRow(1) = A/dr^2 - A/3/dr/rVec(2);
secondRow(2) = - 2*A/dr^2 - A/2/dr/rVec(2);
secondRow(3) = -A/dr^2 + A/dr/rVec(2);
secondRow(4) = -A /dr^2 + A/dr/rVec(2);
secondRow(5) = A/6/dr/rVec(2);

FDM(2,:) = secondRow; %Checked

for idx = 3: (nNode+1)-2
   FDM(idx,idx-2:idx+2) = genRow(idx,A,rVec,dr);
end


%Second Last Row //this is the neumann condition
SLRow = zeros(1,5);
SLRow(1) = -A/12/dr^2 - A/12/dr/rVec(end-1); %need to subtract 2 to account
SLRow(2) = A/3/dr^2 + A/2/dr/rVec(end-1);
SLRow(3) = A/2/dr^2 - 3*A/2/dr/rVec(end-1);
SLRow(4) = - 5*A/3/dr^2 + 5*A/6/dr/rVec(end-1);
SLRow(5) = 11*A/12/dr^2 + A/4/dr/rVec(end-1); %chedcked, sums to zero; checked against mathematica
FDM(end-1,end-4:end) = SLRow;

%Last Row
lastRow = zeros(1,5);
lastRow(1) = -A/12/dr^2;
lastRow(2) = A/3/dr^2;
lastRow(3) = A/2/dr^2;
lastRow(4) = - 5*A/3/dr^2; % - H*R*T*km/epsilon/rVec(end);
lastRow(5) = 11*A/12/dr^2;
FDM(end,end-4:end) = lastRow;

BMat = zeros(nNode+1);
BMat(1:nNode,1:nNode) = eye(nNode);
BMat(end,end-1) = 1;


HMat = zeros(nNode+1);
HMat(end,end-1) = 1;
rGhost = rVec(end);

== matlab function Xe_Model_Redo_June_26/Graphite /Graphite Region 2/Graphite Stringer/Generate FDM Matrix  ==
  data: FDM output; HMat output; BMat output; r0 input; D_g input; epsilon input; rGhost output
function [FDM,HMat,BMat,rGhost]= genMat(r0,D_g,epsilon)

%SETTINGS
%Don't forget to change the value in the blocks:
%%INJECTION VECTOR
%%RHS IDX
nNode = 20;
%%%%%%

%#codegen

%r0 = 0.01454; %graphite stringer radius
dr = r0/(nNode-1); %we have nNode-1 internal 'posts'
rVec = horzcat(linspace(0,r0 ,nNode),r0+dr); %positions of each node, include ghost node
FDM = zeros(nNode+1);

%D_g = 2.37E-9;
%epsilon = 0.1;

A= D_g/epsilon;
 

topRow = zeros(1,nNode+1);
topRow(1) = - (5*A) / (4*dr^2);
topRow(2) = A / dr^2;
topRow(3) = A / (4*dr^2);

FDM(1,:) = topRow; %From Prior Code`

%Second Row
secondRow = zeros(1,nNode+1);

secondRow(1) = A/dr^2 - A/3/dr/rVec(2);
secondRow(2) = - 2*A/dr^2 - A/2/dr/rVec(2);
secondRow(3) = -A/dr^2 + A/dr/rVec(2);
secondRow(4) = -A /dr^2 + A/dr/rVec(2);
secondRow(5) = A/6/dr/rVec(2);

FDM(2,:) = secondRow; %Checked

for idx = 3: (nNode+1)-2
   FDM(idx,idx-2:idx+2) = genRow(idx,A,rVec,dr);
end


%Second Last Row //this is the neumann condition
SLRow = zeros(1,5);
SLRow(1) = -A/12/dr^2 - A/12/dr/rVec(end-1); %need to subtract 2 to account
SLRow(2) = A/3/dr^2 + A/2/dr/rVec(end-1);
SLRow(3) = A/2/dr^2 - 3*A/2/dr/rVec(end-1);
SLRow(4) = - 5*A/3/dr^2 + 5*A/6/dr/rVec(end-1);
SLRow(5) = 11*A/12/dr^2 + A/4/dr/rVec(end-1); %chedcked, sums to zero; checked against mathematica
FDM(end-1,end-4:end) = SLRow;

%Last Row
lastRow = zeros(1,5);
lastRow(1) = -A/12/dr^2;
lastRow(2) = A/3/dr^2;
lastRow(3) = A/2/dr^2;
lastRow(4) = - 5*A/3/dr^2;% - H*R*T*km/epsilon/rVec(end);
lastRow(5) = 11*A/12/dr^2;
FDM(end,end-4:end) = lastRow;

BMat = zeros(nNode+1);
BMat(1:nNode,1:nNode) = eye(nNode);
BMat(end,end-1) = 1;


HMat = zeros(nNode+1);
HMat(end,end-1) = 1;
rGhost = rVec(end);

== matlab function Xe_Model_Redo_June_26/Graphite /Graphite Region 1/Graphite Stringer/Generate FDM Matrix  ==
  data: FDM output; HMat output; BMat output; r0 input; D_g input; epsilon input; rGhost output
function [FDM,HMat,BMat,rGhost]= genMat(r0,D_g,epsilon)

%SETTINGS
%Don't forget to change the value in the blocks:
%%INJECTION VECTOR
%%RHS IDX
nNode = 20;
%%%%%%

%#codegen

%r0 = 0.01454; %graphite stringer radius
dr = r0/(nNode-1); %we have nNode-1 internal 'posts'
rVec = horzcat(linspace(0,r0 ,nNode),r0+dr); %positions of each node, include ghost node
FDM = zeros(nNode+1);

%D_g = 2.37E-9;
%epsilon = 0.1;

A= D_g/epsilon;
 

topRow = zeros(1,nNode+1);
topRow(1) = - (5*A) / (4*dr^2);
topRow(2) = A / dr^2;
topRow(3) = A / (4*dr^2);

FDM(1,:) = topRow; %From Prior Code`

%Second Row
secondRow = zeros(1,nNode+1);

secondRow(1) = A/dr^2 - A/3/dr/rVec(2);
secondRow(2) = - 2*A/dr^2 - A/2/dr/rVec(2);
secondRow(3) = -A/dr^2 + A/dr/rVec(2);
secondRow(4) = -A /dr^2 + A/dr/rVec(2);
secondRow(5) = A/6/dr/rVec(2);

FDM(2,:) = secondRow; %Checked

for idx = 3: (nNode+1)-2
   FDM(idx,idx-2:idx+2) = genRow(idx,A,rVec,dr);
end


%Second Last Row //this is the neumann condition
SLRow = zeros(1,5);
SLRow(1) = -A/12/dr^2 - A/12/dr/rVec(end-1); %need to subtract 2 to account
SLRow(2) = A/3/dr^2 + A/2/dr/rVec(end-1);
SLRow(3) = A/2/dr^2 - 3*A/2/dr/rVec(end-1);
SLRow(4) = - 5*A/3/dr^2 + 5*A/6/dr/rVec(end-1);
SLRow(5) = 11*A/12/dr^2 + A/4/dr/rVec(end-1); %chedcked, sums to zero; checked against mathematica
FDM(end-1,end-4:end) = SLRow;

%Last Row
lastRow = zeros(1,5);
lastRow(1) = -A/12/dr^2;
lastRow(2) = A/3/dr^2;
lastRow(3) = A/2/dr^2;
lastRow(4) = - 5*A/3/dr^2;% - H*R*T*km/epsilon/rVec(end);
lastRow(5) = 11*A/12/dr^2;
FDM(end,end-4:end) = lastRow;

BMat = zeros(nNode+1);
BMat(1:nNode,1:nNode) = eye(nNode);
BMat(end,end-1) = 1;


HMat = zeros(nNode+1);
HMat(end,end-1) = 1;
rGhost = rVec(end);
